simulink model "simu_2"  (R2013b)
settings: Solver=ode45  StartTime=0.0  StopTime=3  FixedStep=0.01  RelTol=1e-3
values from neighbouring files (symbols this model uses):
  am = 1    [main.m]
  ap = -6    [main.m]
  cm = 1    [main.m]
  cp = 1    [main.m]
  dxm0 = 0    [main.m]
  dxp0 = 0    [main.m]
  km = 1    [main.m]
  kp = 1    [main.m]
  theta0 = [0 0 0 0 0]'    [main.m]
  xm0 = 0    [main.m]
  xp0 = 0    [main.m]
settings Model: Creator=andreas  LastModifiedBy=andreas
settings DebuggingCC: UnderspecifiedInitializationDetection=Simplified  MergeDetectMultiDrivingBlocksExec=error  SolverPrmCheckMsg=none  FrameProcessingCompatibilityMsg=error
settings GRTTargetCC: CodeReplacementLibrary=C89/C90 (ANSI)

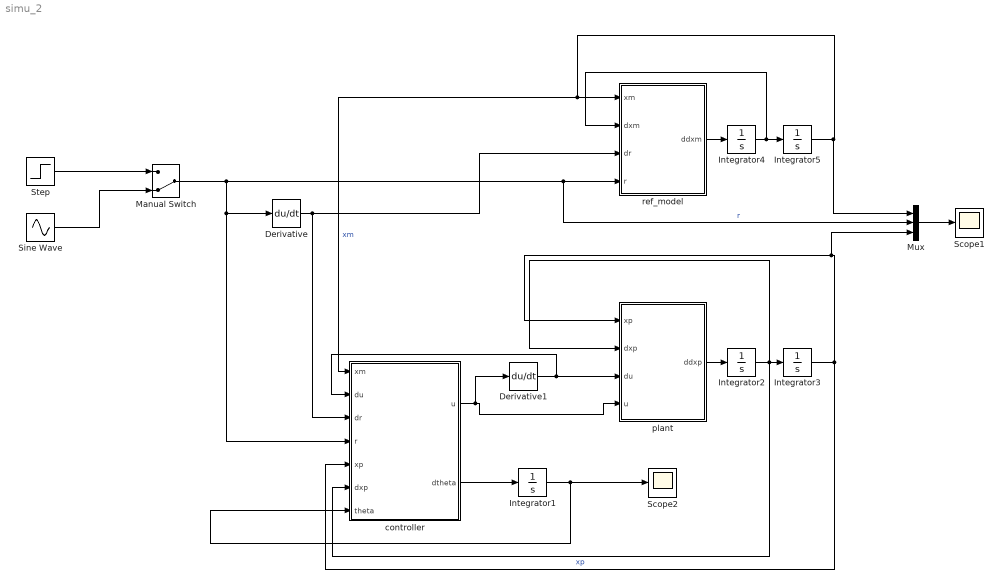
== system simu_2 ==
  Derivative : Derivative
  Derivative1 : Derivative
  Integrator1 : Integrator  InitialCondition=theta0
  Integrator2 : Integrator  InitialCondition=dxp0
  Integrator3 : Integrator  InitialCondition=xp0
  Integrator4 : Integrator  InitialCondition=dxm0
  Integrator5 : Integrator  InitialCondition=xm0
  Manual Switch : ManualSwitch  CurrentSetting=0
  Mux : Mux  Inputs=3
  Scope1 : Scope
      settings: ShowLegends=on  YMin=0  YMax=2.5
  Scope2 : Scope
      settings: ShowLegends=on  YMin=-0.15  YMax=0.25  SaveName=ScopeData2
  Sine Wave : Sin  Amplitude=4  Frequency=2*pi/10  SampleTime=0
  Step : Step  SampleTime=0
  controller : MATLAB Function  TreatAsAtomicUnit=on
      settings: PermitHierarchicalResolution=ParametersOnly
  plant : MATLAB Function  TreatAsAtomicUnit=on
      settings: PermitHierarchicalResolution=ParametersOnly
  ref_model : MATLAB Function  TreatAsAtomicUnit=on
      settings: PermitHierarchicalResolution=ParametersOnly
  wires:
  controller/1(u) -> Derivative1/1, plant/4(u)
  controller/2(dtheta) -> Integrator1/1
  plant/1(ddxp) -> Integrator2/1
  Integrator2/1 -> controller/6(dxp), plant/2(dxp), Integrator3/1
  ref_model/1(ddxm) -> Integrator4/1
  Mux/1 -> Scope1/1
  Step/1 -> Manual Switch/1
  Sine Wave/1 -> Manual Switch/2
  Integrator4/1 -> ref_model/2(dxm), Integrator5/1
  Integrator1/1 -> Scope2/1, controller/7(theta)
  Integrator5/1 -> Mux/1, controller/1(xm), ref_model/1(xm)  "xm"
  Manual Switch/1 -> Derivative/1, controller/4(r), Mux/2, ref_model/4(r)  "r"
  Derivative/1 -> controller/3(dr), ref_model/3(dr)
  Derivative1/1 -> controller/2(du), plant/3(du)
  Integrator3/1 -> Mux/3, plant/1(xp), controller/5(xp)  "xp"

== matlab function simu_2/ref_model ==
  data: xm input; dxm input; dr input; r input; km parameter; cm parameter; am parameter; ddxm output
function ddxm = ref_model(xm, dxm, dr, r, km, cm, am)
%#codegen

ddxm = km*dr + cm*km*r - (am+cm)*dxm - am*cm*xm;

== matlab function simu_2/controller ==
  data: xm input; du input; u output; dr input; r input; xp input; dxp input; theta input; dtheta output; gamma parameter
function [u, dtheta] = controller(xm, du, dr, r, xp, dxp, theta, gamma)
%#codegen

e = xp - xm;

phi = [dr, r, dxp, xp, du]';

u = theta'*phi;

dtheta = -gamma*phi*e;

== matlab function simu_2/plant ==
  data: xp input; dxp input; du input; u input; kp parameter; cp parameter; ddxp output; ap parameter
function ddxp = plant(xp, dxp, du, u, kp, cp, ap)
%#codegen

ddxp = kp*du + cp*kp*u - (ap+cp)*dxp + ap*cp*xp;
